simulink model "WheelModel"  (R2024a)
settings: Solver=VariableStepAuto  StartTime=0.0  StopTime=60  RelTol=1e-3
undefined symbols (not defined in the file or in its folder): g, J_p, J_w, K, l, m, omega_max
settings Model: Creator=Jonah  LastModifiedBy=Jonah

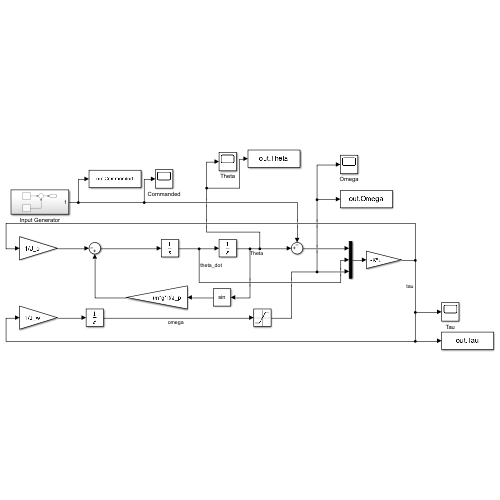
[thumbnail: Simulink's stored preview of the top-level diagram]
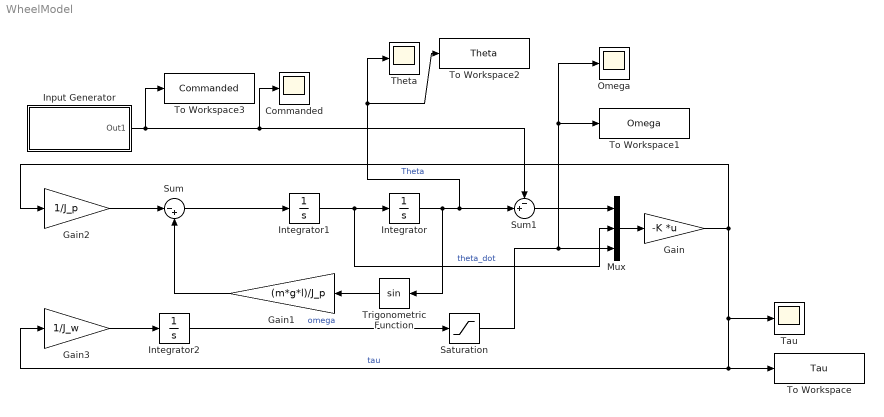
== system WheelModel ==
  Commanded : Scope
  Gain : Gain  Gain=-K  Multiplication=Matrix(K*u)
  Gain1 : Gain  Gain=(m*g*l)/J_p
  Gain2 : Gain  Gain=1/J_p
  Gain3 : Gain  Gain=1/J_w
  Input Generator : Subsystem
  Integrator : Integrator
  Integrator1 : Integrator
  Integrator2 : Integrator
  Mux : Mux  Inputs=3
  Omega : Scope
  Saturation : Saturate  UpperLimit=omega_max  LowerLimit=-omega_max
  Sum : Sum  Inputs=|-+
  Sum1 : Sum  Inputs=-+|
  Tau : Scope
  Theta : Scope
  To Workspace : ToWorkspace  VariableName=Tau  SaveFormat=Timeseries  SampleTime=-1
  To Workspace1 : ToWorkspace  VariableName=Omega  SaveFormat=Timeseries  SampleTime=-1
  To Workspace2 : ToWorkspace  VariableName=Theta  SaveFormat=Timeseries  SampleTime=-1
  To Workspace3 : ToWorkspace  VariableName=Commanded  SaveFormat=Timeseries  SampleTime=-1
  Trigonometric Function : Trigonometry
  wires:
  Mux/1 -> Gain/1
  Sum1/1 -> Mux/1
  Integrator/1 -> Sum1/2, To Workspace2/1, Theta/1, Trigonometric Function/1  "Theta"
  Integrator1/1 -> Mux/2, Integrator/1  "theta_dot"
  Trigonometric Function/1 -> Gain1/1
  Sum/1 -> Integrator1/1
  Gain1/1 -> Sum/2
  Gain2/1 -> Sum/1
  Gain/1 -> Gain2/1, Tau/1, Gain3/1, To Workspace/1  "tau"
  Gain3/1 -> Integrator2/1
  Integrator2/1 -> Saturation/1  "omega"
  Saturation/1 -> To Workspace1/1, Omega/1, Mux/3
  Input Generator/1(Out1) -> To Workspace3/1, Commanded/1, Sum1/1

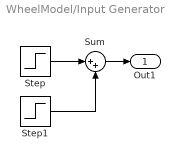
== system WheelModel/Input Generator ==
  Step : Step  Before=-1  After=0  SampleTime=0
  Step1 : Step  Time=2  Before=1  After=0  SampleTime=0
  Sum : Sum  Inputs=|++
  Out1 : Outport
  wires:
  Step1/1 -> Sum/2
  Step/1 -> Sum/1
  Sum/1 -> Out1/1
